simulink model "aufgabe_2"  (R2017b)
settings: Solver=VariableStepAuto  StartTime=0.0  StopTime=3  RelTol=1e-3
settings Model: Creator=gurbuz  LastModifiedBy=gurbuz

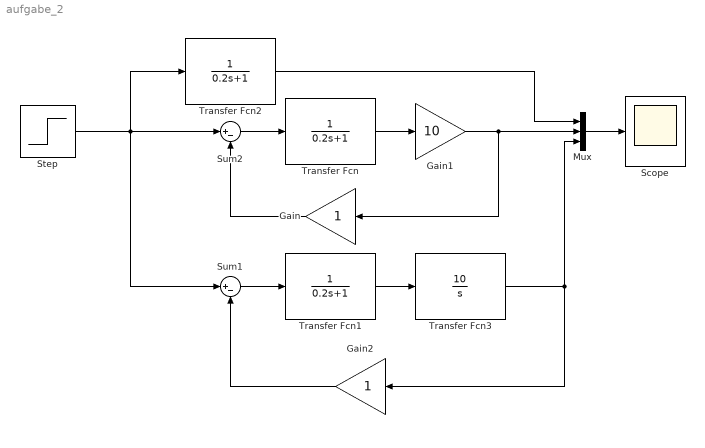
== system aufgabe_2 ==
  Gain : Gain
  Gain1 : Gain  Gain=10
  Gain2 : Gain
  Mux : Mux  Inputs=3
  Scope : Scope
  Step : Step  Time=0  SampleTime=0
  Sum1 : Sum  Inputs=|+-
  Sum2 : Sum  Inputs=|+-
  Transfer Fcn : TransferFcn  Denominator=[0.2 1]
  Transfer Fcn1 : TransferFcn  Denominator=[0.2 1]
  Transfer Fcn2 : TransferFcn  Denominator=[0.2 1]
  Transfer Fcn3 : TransferFcn  Numerator=[10]  Denominator=[1 0]
  wires:
  Step/1 -> Sum1/1, Sum2/1, Transfer Fcn2/1
  Sum2/1 -> Transfer Fcn/1
  Transfer Fcn/1 -> Gain1/1
  Gain1/1 -> Mux/2, Gain/1
  Gain/1 -> Sum2/2
  Sum1/1 -> Transfer Fcn1/1
  Transfer Fcn1/1 -> Transfer Fcn3/1
  Transfer Fcn3/1 -> Mux/3, Gain2/1
  Gain2/1 -> Sum1/2
  Transfer Fcn2/1 -> Mux/1
  Mux/1 -> Scope/1
